simulink model "visualization"  (R2021a)
settings: Solver=FixedStepAuto  StartTime=0.0  StopTime=inf  FixedStep=0.04  RelTol=1e-3
InitFcn:
  | run initialize.m
StopFcn:
  | run save_result.m
libraries: dspbuff3 x2, robotlib x1
settings Model: EnablePacing=on  Creator=rocky  LastModifiedBy=jeremy

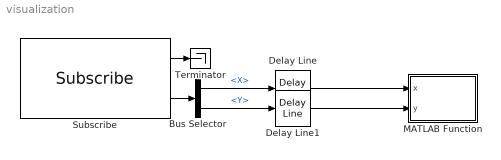
== system visualization ==
  Bus Selector : BusSelector  OutputSignals=Pose.Position.X,Pose.Position.Y
  Delay Line : dspbuff3/Delay Line  siz=40  ic=0  directfeed=off  enable_output=off  hold_output=off  OutputFrames=off
      settings: SourceProductBaseCode=DS
  Delay Line1 : dspbuff3/Delay Line  siz=40  ic=0  directfeed=off  enable_output=off  hold_output=off  OutputFrames=off
      settings: SourceProductBaseCode=DS
  MATLAB Function : MATLAB Function  TreatAsAtomicUnit=on
  Subscribe : robotlib/Subscribe  topicSource=Select from ROS network  topic=/mavros/local_position/pose  messageType=geometry_msgs/PoseStamped  SampleTime=-1  legacyBusStruct=off  messageQueueLength=1
  Terminator : Terminator
  wires:
  Bus Selector/2 -> Delay Line1/1  "<Y>"
  Bus Selector/1 -> Delay Line/1  "<X>"
  Delay Line/1 -> MATLAB Function/1(x)
  Delay Line1/1 -> MATLAB Function/2(y)
  Subscribe/2 -> Bus Selector/1
  Subscribe/1 -> Terminator/1

== matlab function visualization/MATLAB Function ==
  data: x input; y input
function traj_plot(x,y)

    figure(1);

    plot(x(end),y(end),'.','MarkerSize',20,'Color',[0 0.4470 0.7410]);
    hold on
    plot(x,y,'-','Color',[0 0.4470 0.7410],'LineWidth',1.5);
    
    xlim([-5 5]);
    ylim([-5 5]);
    axis equal
    
    hold off

end
